simulink model "thermal_model"  (R2023a)
settings: Solver=FixedStepDiscrete  StartTime=0.0  StopTime=10.0  FixedStep=ThermalModel_Ts  RelTol=1e-3  EnableMultiTasking=on
model workspace (MAT data in the model file):
  ThermalModel_Ts = Simulink.Parameter
  ThermalModel_Ts.Value = 0.01
  ThermalModel_Ts.DataType = 'auto'
  ThermalModel_Ts.DocUnits = 's'
  ThermalModel_Ts.Complexity = 'real'
  ThermalModel_Ts.Dimensions = [1 1]
settings Model: DataDictionary=EmbeddedBoardDD.sldd  Creator=ascalzo  LastModifiedBy=upattacini
settings SolverCC: AllowMultiTaskInputOutput=on  AutoInsertRateTranBlk=on  InsertRTBMode=Never (minimum delay)
settings DataIOCC: SaveOutput=off  SignalLogging=off  DSMLogging=off  SaveTime=off  ReturnWorkspaceOutputs=off
settings OptimizationCC: DefaultParameterBehavior=Inlined  DefaultUnderspecifiedDataType=single  StrengthReduction=on  PassReuseOutputArgsAs=Individual arguments  ZeroExternalMemoryAtStartup=off  ZeroInternalMemoryAtStartup=off  OptimizeBlockOrder=speed  OptimizationPriority=Speed  OptimizationCustomize=off  MultiThreadedLoops=on  EfficientTunableParamExpr=on
settings DebuggingCC: ParameterPrecisionLossMsg=none  UnconnectedInputMsg=warning  UnconnectedOutputMsg=warning  UnconnectedLineMsg=warning
settings HardwareCC: ProdBitPerPointer=32  ProdBitPerSizeT=32  ProdBitPerPtrDiffT=32  ProdLargestAtomicInteger=Long  ProdLargestAtomicFloat=Double  ProdWordSize=32  ProdHWDeviceType=ARM Compatible->ARM Cortex-M
settings ModelReferenceCC: UpdateModelReferenceTargets=Force  EnableRefExpFcnMdlSchedulingChecks=on  ModelReferenceNumInstancesAllowed=Single
settings SFSimCC: MATLABDynamicMemAlloc=off
settings RTWCC: Description=Embedded Coder  SystemTargetFile=ert.tlc  GenCodeOnly=on  PackageGeneratedCodeAndArtifacts=on  PackageName=filter_current  TemplateMakefile=ert_default_tmf  TargetLang=C++  DLArmComputeVersion=19.05
settings CodeAppCC: ForceParamTrailComments=on  IgnoreCustomStorageClasses=off  OperatorAnnotations=on  SimulinkDataObjDesc=on  SFDataObjDesc=on  InsertBlockDesc=on
settings ERTTargetCC: TargetLangStandard=C++03 (ISO)  CodeReplacementLibrary=ARM Cortex-M,iCubTech  GenerateSampleERTMain=on  InlinedParameterPlacement=NonHierarchical  RootIOFormat=Structure reference  ERTCustomFileTemplate=example_file_process.tlc

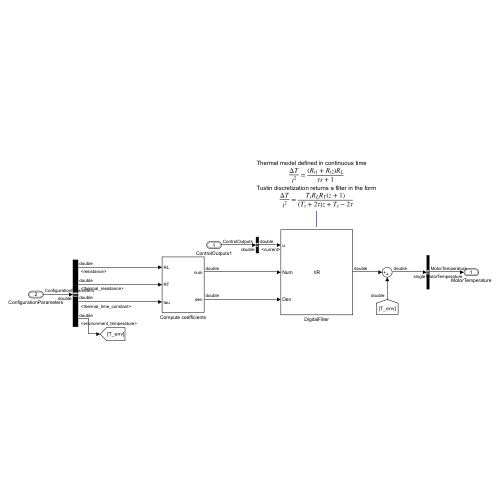
[thumbnail: Simulink's stored preview of the top-level diagram]
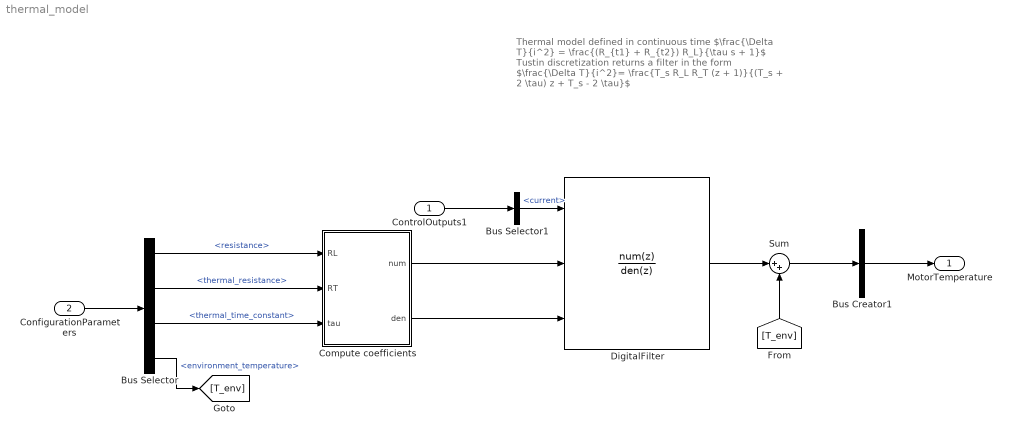
== system thermal_model ==
  note: Thermal model defined in continuous time
      | $\frac{\Delta T}{i^2} = \frac{(R_{t1} + R_{t2}) R_L}{\tau s + 1}$
      | Tustin discretization returns a filter in the form
      | $\frac{\Delta T}{i^2}= \frac{T_s R_L R_T (z + 1)}{(T_s + 2 \tau) z + T_s - 2 \tau}$
  ControlOutputs1 : Inport  OutDataTypeStr=Bus: ControlOutputs  BusOutputAsStruct=on
  ConfigurationParameters : Inport  Port=2  OutDataTypeStr=Bus: ConfigurationParameters  BusOutputAsStruct=on
  Bus Creator1 : BusCreator  Inputs=1  OutDataTypeStr=Bus: MotorTemperature  NonVirtualBus=on
      settings: InheritFromInputs=off
  Bus Selector : BusSelector  OutputSignals=motorconfig.resistance,motorconfig.thermal_resistance,motorconfig.thermal_time_constant,environment_temperature
  Bus Selector1 : BusSelector  OutputSignals=Iq_fbk.current
  Compute coefficients : Subsystem
  DigitalFilter : DiscreteFilter  NumeratorSource=Input port  Numerator="[0.02685   0.02685]"  DenominatorSource=Input port  Denominator=[1 -0.9999629]  FilterStructure=Direct form II transposed  SampleTime=ThermalModel_Ts  a0EqualsOne=on  OutDataTypeStr=Inherit: Same as input
      settings: InputPortMap=u0,p1,p3
  Sum : Sum  Inputs=|++
  MotorTemperature : Outport  OutDataTypeStr=Bus: MotorTemperature  BusOutputAsStruct=on
  wires:
  Bus Creator1/1 -> MotorTemperature/1
  DigitalFilter/1 -> Sum/1
  Bus Selector/2 -> Compute coefficients/2(RT)  "<thermal_resistance>"
  Bus Selector/1 -> Compute coefficients/1(RL)  "<resistance>"
  ConfigurationParameters/1 -> Bus Selector/1
  Bus Selector/4 -> [T_env]  "<environment_temperature>"
  Compute coefficients/2(den) -> DigitalFilter/3
  Compute coefficients/1(num) -> DigitalFilter/2
  Bus Selector1/1 -> DigitalFilter/1  "<current>"
  Bus Selector/3 -> Compute coefficients/3(tau)  "<thermal_time_constant>"
  Sum/1 -> Bus Creator1/1
  [T_env] -> Sum/2
  ControlOutputs1/1 -> Bus Selector1/1

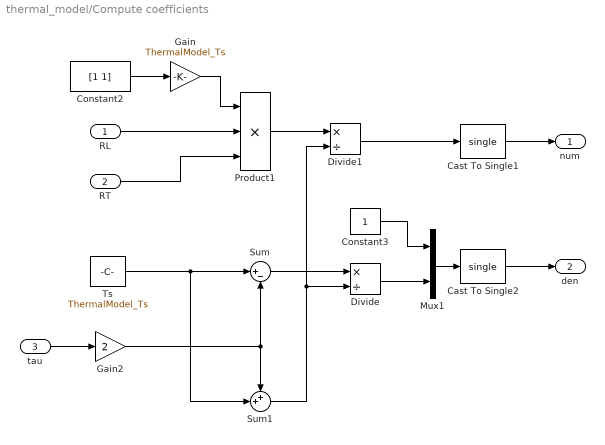
== system thermal_model/Compute coefficients ==
  RL : Inport
  RT : Inport  Port=2
  tau : Inport  Port=3
  Cast To Single1 : DataTypeConversion  OutDataTypeStr=single  SaturateOnIntegerOverflow=off  RndMeth=Floor
  Cast To Single2 : DataTypeConversion  OutDataTypeStr=single  SaturateOnIntegerOverflow=off  RndMeth=Floor
  Constant2 : Constant  Value=[1 1]  OutDataTypeStr=single  SampleTime=ThermalModel_Ts
  Constant3 : Constant  OutDataTypeStr=single  SampleTime=ThermalModel_Ts
  Divide : Product  Inputs=*/
  Divide1 : Product  Inputs=*/
  Gain : Gain  Gain=ThermalModel_Ts
  Gain2 : Gain  Gain=2
  Mux1 : Mux  Inputs=2
  Product1 : Product  Inputs=3
  Sum : Sum  Inputs=|+-
  Sum1 : Sum  Inputs=++|
  Ts : Constant  Value=ThermalModel_Ts  OutDataTypeStr=single  SampleTime=ThermalModel_Ts
  num : Outport
  den : Outport  Port=2
  wires:
  Mux1/1 -> Cast To Single2/1
  Sum1/1 -> Divide/2, Divide1/2
  Product1/1 -> Divide1/1
  Divide1/1 -> Cast To Single1/1
  Gain/1 -> Product1/1
  tau/1 -> Gain2/1
  Constant3/1 -> Mux1/1
  RL/1 -> Product1/2
  Ts/1 -> Sum1/2, Sum/1
  Sum/1 -> Divide/1
  Gain2/1 -> Sum1/1, Sum/2
  Constant2/1 -> Gain/1
  Divide/1 -> Mux1/2
  Cast To Single2/1 -> den/1
  RT/1 -> Product1/3
  Cast To Single1/1 -> num/1
